simulink model "two_bus_linear"  (R2020b)
settings: Solver=VariableStepAuto  StartTime=0.0  StopTime=1  RelTol=1e-3
libraries: powerlib x41
settings Model: Creator=tmcnama2  LastModifiedBy=tmcnama2

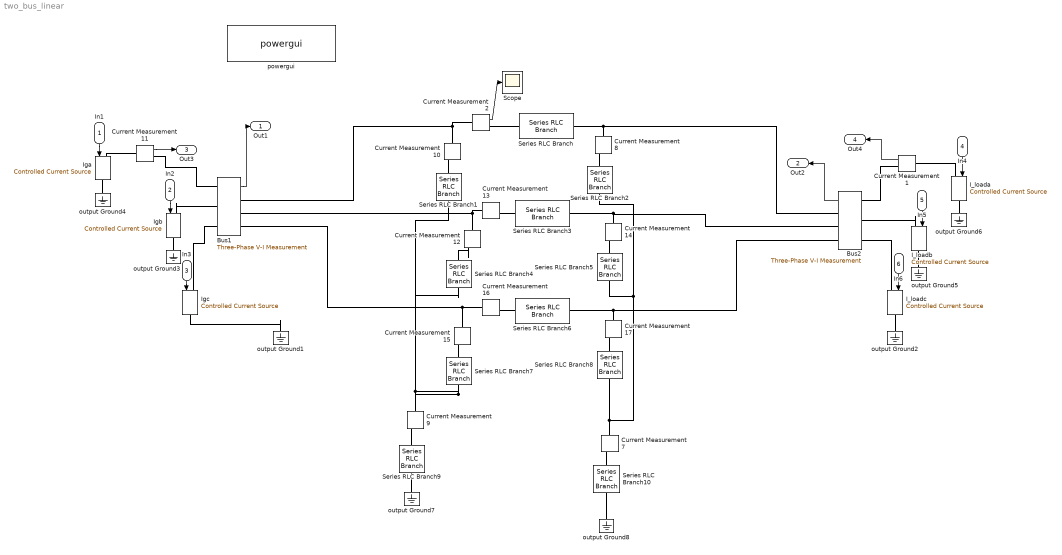
== system two_bus_linear ==
  In1 : Inport
  In2 : Inport  Port=2
  In3 : Inport  Port=3
  In4 : Inport  Port=4
  In5 : Inport  Port=5
  In6 : Inport  Port=6
  Bus1 : powerlib/Measurements/Three-Phase V-I Measurement  VoltageMeasurement=phase-to-ground  SetLabelV=off  LabelV=VB1  Vpu=off  VpuLL=off  CurrentMeasurement=no  SetLabelI=off  LabelI=IB1  Ipu=off  Pbase=100e6  Vbase=500e3  OutputType=Complex  PhasorSimulation=off  PSBequivalent=0
  Bus2 : powerlib/Measurements/Three-Phase V-I Measurement  VoltageMeasurement=phase-to-ground  SetLabelV=off  LabelV=VB1  Vpu=off  VpuLL=off  CurrentMeasurement=no  SetLabelI=off  LabelI=IB1  Ipu=off  Pbase=100e6  Vbase=500e3  OutputType=Complex  PhasorSimulation=off  PSBequivalent=0
  Current Measurement{1..2,7..17} (13 alike) : powerlib/Measurements/Current Measurement  PhasorSimulation=off  OutputType=Complex  PSBequivalent=0
  I_loada : powerlib/Electrical Sources/Controlled Current Source  Initialize=on  Source_Type=AC  Amplitude=0  Phase=0  Frequency=0  Measurements=None
  I_loadb : powerlib/Electrical Sources/Controlled Current Source  Initialize=on  Source_Type=AC  Amplitude=0  Phase=0  Frequency=0  Measurements=None
  I_loadc : powerlib/Electrical Sources/Controlled Current Source  Initialize=on  Source_Type=AC  Amplitude=0  Phase=0  Frequency=0  Measurements=None
  Iga : powerlib/Electrical Sources/Controlled Current Source  Initialize=on  Source_Type=AC  Amplitude=0  Phase=0  Frequency=0  Measurements=None
  Igb : powerlib/Electrical Sources/Controlled Current Source  Initialize=on  Source_Type=AC  Amplitude=0  Phase=0  Frequency=0  Measurements=None
  Igc : powerlib/Electrical Sources/Controlled Current Source  Initialize=on  Source_Type=AC  Amplitude=0  Phase=0  Frequency=0  Measurements=None
  Scope : Scope
  Series RLC Branch : powerlib/Elements/Series RLC Branch  LConnTagsString=__new0  RConnTagsString=__new0  BranchType=RL  Resistance=1.2730  Inductance=0.41264  SetiL0=off  InitialCurrent=0  Capacitance=1e-6  Setx0=off  InitialVoltage=0  Measurements=None
  Series RLC Branch{1..2,4..5,7..8} (6 alike) : powerlib/Elements/Series RLC Branch  LConnTagsString=__new0  RConnTagsString=__new0  BranchType=C  Resistance=1.2730  Inductance=0.4126  SetiL0=off  InitialCurrent=0  Capacitance=1.2740e-06/2  Setx0=off  InitialVoltage=0  Measurements=None
  Series RLC Branch10 : powerlib/Elements/Series RLC Branch  LConnTagsString=__new0  RConnTagsString=__new0  BranchType=C  Resistance=1.2730  Inductance=0.4126  SetiL0=off  InitialCurrent=0  Capacitance=5.9379e-06/2  Setx0=off  InitialVoltage=0  Measurements=None
  Series RLC Branch3 : powerlib/Elements/Series RLC Branch  LConnTagsString=__new0  RConnTagsString=__new0  BranchType=RL  Resistance=1.2730  Inductance=0.41264  SetiL0=off  InitialCurrent=0  Capacitance=1e-6  Setx0=off  InitialVoltage=0  Measurements=None
  Series RLC Branch6 : powerlib/Elements/Series RLC Branch  LConnTagsString=__new0  RConnTagsString=__new0  BranchType=RL  Resistance=1.2730  Inductance=0.41264  SetiL0=off  InitialCurrent=0  Capacitance=1e-6  Setx0=off  InitialVoltage=0  Measurements=None
  Series RLC Branch9 : powerlib/Elements/Series RLC Branch  LConnTagsString=__new0  RConnTagsString=__new0  BranchType=C  Resistance=1.2730  Inductance=0.4126  SetiL0=off  InitialCurrent=0  Capacitance=5.9379e-06/2  Setx0=off  InitialVoltage=0  Measurements=None
  output Ground{1..8} (8 alike) : powerlib/Elements/Ground  LConnTagsString=a
  powergui : powerlib/powergui  Priority=1  SimulationMode=Discrete  SampleTime=50e-6  frequency=60  Iterations=50  frequencyindice=0  Pbase=120e6  ErrMax=0.0001  UnitsV=kV  UnitsW=MW  buscounter=0  FunctionMessages=off  echomessages=off  EnableUseOfTLC=off  CurrentSourceSwitches=off  DisableSnubberDevices=off  DisableRonSwitches=off  DisableVfSwitches=off  DisplayEquations=off  AutomaticDiscreteSolvers=off  SolverType=Tustin/Backward Euler (TBE)  Interpol=off  ExternalGateDelay=off  methode=off  Ts=100  x0status=zero  SPID=on  SwTol=0  HookPort=off  NonlinearTolerance=1e-4  nMaxIteration=100  ContinueOnMaxIteration=off  RestoreLinks=warning  ResistiveCurrentMeasurement=off  Frange=[0:2:500]  Ylog=off  Xlog=on  ShowGrid=off  save=off  variable=ZData  structure=0  ZoomFFT=off  StartTime=0.0  cycles=1  DisplayStyle=1  fundamental=60  FreqAxis=off  MaxFrequency=1000  frequencyindicesteady=1  RmsSteady=1  display=off
  Out1 : Outport
  Out2 : Outport  Port=2
  Out3 : Outport  Port=3
  Out4 : Outport  Port=4
  wires:
  In1/1 -> Iga/1
  In2/1 -> Igb/1
  In3/1 -> Igc/1
  In4/1 -> I_loada/1
  In5/1 -> I_loadb/1
  In6/1 -> I_loadc/1
  Bus1/1 -> Out1/1
  Bus2/1 -> Out2/1
  Current Measurement11/1 -> Out3/1
  Current Measurement1/1 -> Out4/1
  Current Measurement2/1 -> Scope/1
  connections:
  output Ground1/LConn1 -- Igc/RConn1
  output Ground2/LConn1 -- I_loadc/RConn1
  Igb/LConn1 -- Bus1/LConn2
  Igc/LConn1 -- Bus1/LConn3
  Series RLC Branch/RConn1 -- Bus2/RConn1 -- Current Measurement8/LConn1
  I_loadb/LConn1 -- Bus2/LConn2
  I_loadc/LConn1 -- Bus2/LConn3
  Current Measurement11/RConn1 -- Bus1/LConn1
  Current Measurement11/LConn1 -- Iga/LConn1
  Current Measurement1/RConn1 -- Bus2/LConn1
  Current Measurement1/LConn1 -- I_loada/LConn1
  output Ground3/LConn1 -- Igb/RConn1
  output Ground5/LConn1 -- I_loadb/RConn1
  output Ground6/LConn1 -- I_loada/RConn1
  output Ground4/LConn1 -- Iga/RConn1
  Current Measurement12/LConn1 -- Current Measurement13/LConn1 -- Bus1/RConn2
  Current Measurement15/LConn1 -- Bus1/RConn3 -- Current Measurement16/LConn1
  output Ground7/LConn1 -- Series RLC Branch9/RConn1
  output Ground8/LConn1 -- Series RLC Branch10/RConn1
  Series RLC Branch5/RConn1 -- Current Measurement7/LConn1 -- Series RLC Branch8/RConn1 -- Series RLC Branch2/RConn1
  Series RLC Branch7/RConn1 -- Current Measurement9/LConn1 -- Series RLC Branch4/RConn1 -- Series RLC Branch1/RConn1
  Series RLC Branch3/RConn1 -- Bus2/RConn2 -- Current Measurement14/LConn1
  Series RLC Branch6/RConn1 -- Bus2/RConn3 -- Current Measurement17/LConn1
  Current Measurement10/LConn1 -- Current Measurement2/LConn1 -- Bus1/RConn1
  Current Measurement16/RConn1 -- Series RLC Branch6/LConn1
  Current Measurement8/RConn1 -- Series RLC Branch2/LConn1
  Current Measurement12/RConn1 -- Series RLC Branch4/LConn1
  Current Measurement2/RConn1 -- Series RLC Branch/LConn1
  Current Measurement14/RConn1 -- Series RLC Branch5/LConn1
  Current Measurement15/RConn1 -- Series RLC Branch7/LConn1
  Current Measurement10/RConn1 -- Series RLC Branch1/LConn1
  Current Measurement9/RConn1 -- Series RLC Branch9/LConn1
  Current Measurement7/RConn1 -- Series RLC Branch10/LConn1
  Current Measurement13/RConn1 -- Series RLC Branch3/LConn1
  Current Measurement17/RConn1 -- Series RLC Branch8/LConn1
